simulink library "xpcseriallib"  (Simulink 7.7)
settings: Solver=FixedStepDiscrete  StartTime=0.0  StopTime=inf  RelTol=1e-3
undefined symbols (not defined in the file or in its folder): baddr1, baddr2, mbaseserialbinmask, mbaseserialmask, mdiamondemeraldfifomask, mdiamondemeraldmask, mmodemcontrol, mqua2mask, mquafifomask, mquamask, mrs232
libraries: xpcseriallib x614, xpclib x16, simulink x12
(part 2 of 7)

== system xpcseriallib/Diamond/Emerald-MM8  ==
  Diamond Emerald-MM8 Serial : Subsystem  InitFcn=mdiamondemeraldmask(4,8)  mask(RS232 Send Receive){group=Receive Setup, port=1, irqnum=5, saddr1=0x200, baud1=115200, parity1=None, ndata1=8, nstop1=1, fifomode1=16 deep, rlevel1=1, automode1=on, xmtfifosize1=1024, xmtdatatype1=8 bit uint null terminated, rcvfifosize1=1024, rcvmaxread1=1024, rcvminread1=1, rcvusedelim1=on, rcvdelim1=13, rcvdatatype1=count+16 bit uint, rcvsampletime1=-1, baud2=115200, parity2=None, ndata2=8, nstop2=1, fifomode2=16 deep, rlevel2=1, automode2=on, xmtfifosize2=1024, xmtdatatype2=8 bit uint null terminated, rcvfifosize2=1024, rcvmaxread2=1024, rcvminread2=1, rcvusedelim2=on, rcvdelim2=13, rcvdatatype2=count+16 bit uint, rcvsampletime2=-1, baud3=115200, parity3=None, ndata3=8, nstop3=1, fifomode3=16 deep, rlevel3=1, automode3=on, xmtfifosize3=1024, xmtdatatype3=8 bit uint null terminated, rcvfifosize3=1024, rcvmaxread3=1024, rcvminread3=1, rcvusedelim3=on, rcvdelim3=13, rcvdatatype3=count+16 bit uint, rcvsampletime3=-1, baud4=115200, parity4=None, ndata4=8, nstop4=1, fifomode4=16 deep, rlevel4=1, automode4=on, xmtfifosize4=1024, xmtdatatype4=8 bit uint null terminated, rcvfifosize4=1024, rcvmaxread4=1024, rcvminread4=1, rcvusedelim4=on, rcvdelim4=13, rcvdatatype4=count+16 bit uint, rcvsampletime4=-1, baud5=115200, parity5=None, ndata5=8, nstop5=1, fifomode5=16 deep, rlevel5=1, automode5=on, xmtfifosize5=1024, xmtdatatype5=8 bit uint null terminated, rcvfifosize5=1024, rcvmaxread5=1024, rcvminread5=1, rcvusedelim5=on, rcvdelim5=13, rcvdatatype5=count+16 bit uint, rcvsampletime5=-1, baud6=115200, parity6=None, ndata6=8, nstop6=1, fifomode6=16 deep, rlevel6=1, automode6=on, xmtfifosize6=1024, xmtdatatype6=8 bit uint null terminated, rcvfifosize6=1024, rcvmaxread6=1024, rcvminread6=1, rcvusedelim6=on, rcvdelim6=13, rcvdatatype6=count+16 bit uint, rcvsampletime6=-1, baud7=115200, parity7=None, ndata7=8, nstop7=1, fifomode7=16 deep, rlevel7=1, automode7=on, xmtfifosize7=1024, xmtdatatype7=8 bit uint null terminated, rcvfifosize7=1024, rcvmaxread7=1024, rcvminread7=1, rcvusedelim7=on, rcvdelim7=13, rcvdatatype7=count+16 bit uint, rcvsampletime7=-1, baud8=115200, parity8=None, ndata8=8, nstop8=1, fifomode8=16 deep, rlevel8=1, automode8=on, xmtfifosize8=1024, xmtdatatype8=8 bit uint null terminated, rcvfifosize8=1024, rcvmaxread8=1024, rcvminread8=1, rcvusedelim8=on, rcvdelim8=13, rcvdatatype8=count+16 bit uint, rcvsampletime8=-1}
      mask prompts: group "Parameter group:"; port "Port to modify:"; irqnum "IRQ number:"; saddr1 "Base address:"; baud1 "Baud rate:"; parity1 "Parity:"; ndata1 "Data bits:"; nstop1 "Stop bits:"; fifomode1 "Hardware FIFO size:"; rlevel1 "Receive FIFO interrupt level:"; automode1 "Auto RTS/CTS:"; xmtfifosize1 "Transmit software FIFO size:"; xmtdatatype1 "Transmit FIFO data type:"; rcvfifosize1 "Receive software FIFO size:"; rcvmaxread1 "Receive maximum read:"; rcvminread1 "Receive minimum read:"; rcvusedelim1 "Read to delimiter:"; rcvdelim1 "Delimiter:"; rcvdatatype1 "Receive data type:"; rcvsampletime1 "Receive SampleTime:"; baud2 "Baud rate:"; parity2 "Parity:"; ndata2 "Data bits:"; nstop2 "Stop bits:"; fifomode2 "Hardware FIFO size:"; rlevel2 "Receive FIFO interrupt level:"; automode2 "Auto RTS/CTS:"; xmtfifosize2 "Transmit software FIFO size:"; xmtdatatype2 "Transmit FIFO data type:"; rcvfifosize2 "Receive software FIFO size:"; rcvmaxread2 "Receive maximum read:"; rcvminread2 "Receive minimum read:"; rcvusedelim2 "Read to delimiter:"; rcvdelim2 "Delimiter:"; rcvdatatype2 "Receive data type:"; rcvsampletime2 "Receive SampleTime:"; baud3 "Baud rate:"; parity3 "Parity:"; ndata3 "Data bits:"; nstop3 "Stop bits:"; fifomode3 "Hardware FIFO size:"; rlevel3 "Receive FIFO interrupt level:"; automode3 "Auto RTS/CTS:"; xmtfifosize3 "Transmit software FIFO size:"; xmtdatatype3 "Transmit fifo data type:"; rcvfifosize3 "Receive software FIFO size:"; rcvmaxread3 "Receive maximum read:"; rcvminread3 "Receive minimum read:"; rcvusedelim3 "Read to delimiter:"; rcvdelim3 "Delimiter:"; rcvdatatype3 "Receive data type:"; rcvsampletime3 "Receive SampleTime:"; baud4 "Baud rate:"; parity4 "Parity:"; ndata4 "Data bits:"; nstop4 "Stop bits:"; fifomode4 "Hardware FIFO size:"; rlevel4 "Receive FIFO interrupt level:"; automode4 "Auto RTS/CTS:"; xmtfifosize4 "Transmit software FIFO size:"; xmtdatatype4 "Transmit FIFO data type:"; rcvfifosize4 "Receive software FIFO size:"; rcvmaxread4 "Receive maximum read:"; rcvminread4 "Receive minimum read:"; rcvusedelim4 "Read to delimiter:"; rcvdelim4 "Delimiter:"; rcvdatatype4 "Receive data type:"; rcvsampletime4 "Receive SampleTime:"; baud5 "Baud rate:"; parity5 "Parity:"; ndata5 "Data bits:"; nstop5 "Stop bits:"; fifomode5 "Hardware FIFO size:"; rlevel5 "Receive FIFO interrupt level:"; automode5 "Auto RTS/CTS:"; xmtfifosize5 "Transmit software FIFO size:"; xmtdatatype5 "Transmit FIFO data type:"; rcvfifosize5 "Receive software FIFO size:"; rcvmaxread5 "Receive maximum read:"; rcvminread5 "Receive minimum read:"; rcvusedelim5 "Read to delimiter:"; rcvdelim5 "Delimiter:"; rcvdatatype5 "Receive data type:"; rcvsampletime5 "Receive SampleTime:"; baud6 "Baud rate:"; parity6 "Parity:"; ndata6 "Data bits:"; nstop6 "Stop bits:"; fifomode6 "Hardware FIFO size:"; rlevel6 "Receive FIFO interrupt level:"; automode6 "Auto RTS/CTS:"; xmtfifosize6 "Transmit software FIFO size:"; xmtdatatype6 "Transmit FIFO data type:"; rcvfifosize6 "Receive software FIFO size:"; rcvmaxread6 "Receive maximum read:"; rcvminread6 "Receive minimum read:"; rcvusedelim6 "Read to delimiter:"; rcvdelim6 "Delimiter:"; rcvdatatype6 "Receive data type:"; rcvsampletime6 "Receive SampleTime:"; baud7 "Baud rate:"; parity7 "Parity:"; ndata7 "Data bits:"; nstop7 "Stop bits:"; fifomode7 "Hardware FIFO size:"; rlevel7 "Receive FIFO interrupt level:"; automode7 "Auto RTS/CTS:"; xmtfifosize7 "Transmit software FIFO size:"; xmtdatatype7 "Transmit FIFO data type:"; rcvfifosize7 "Receive software FIFO size:"; rcvmaxread7 "Receive maximum read:"; rcvminread7 "Receive minimum read:"; rcvusedelim7 "Read to delimiter:"; rcvdelim7 "Delimiter:"; rcvdatatype7 "Receive data type:"; rcvsampletime7 "Receive SampleTime:"; baud8 "Baud rate:"; parity8 "Parity:"; ndata8 "Data bits:"; nstop8 "Stop bits:"; fifomode8 "Hardware FIFO size:"; rlevel8 "Receive FIFO interrupt level:"; automode8 "Auto RTS/CTS:"; xmtfifosize8 "Transmit software FIFO size:"; xmtdatatype8 "Transmit FIFO data type:"; rcvfifosize8 "Receive software FIFO size:"; rcvmaxread8 "Receive maximum read:"; rcvminread8 "Receive minimum read:"; rcvusedelim8 "Read to delimiter:"; rcvdelim8 "Delimiter:"; rcvdatatype8 "Receive data type:"; rcvsampletime8 "Receive SampleTime:"
      mask help:
      | Diamond Emerald MM-8
      | RS232 Send Receive Subsystem
      mask init:
      | addr = mdiamondemeraldmask( 1, 8 );
      | % addr(1) is base address, not used
      | baddr1 = addr{2};
      | baddr2 = addr{3};
      | baddr3 = addr{4};
      | baddr4 = addr{5};
      | baddr5 = addr{6};
      | baddr6 = addr{7};
      | baddr7 = addr{8};
      | baddr8 = addr{9};
      | istat = addr{10};
      | mdiamondemeraldmask( 3, 8 );
      mask Help: helpview(fullfile(docroot, 'mapfiles', 'xpc.map'), 'Baseboard_Serial_Subsystem')
      mask StyleString: popup(Board Setup|Basic Setup|Transmit Setup|Receive Setup),popup(1|2|3|4|5|6|7|8),edit,popup(0x100|0x140|0x180|0x1c0|0x200|0x240|0x280|0x2c0|0x300|0x340|0x380|0x3c0),popup(115200|57600|38400|19200|9600|4800|2400|1200|600|300|110),popup(None|Even|Odd|Mark|Space),popup(5|6|7|8),popup(1|2),popup(64 deep|16 deep|1 deep),popup(1|quarter full|half full|almost full),checkbox,edit,popup(count+32 bit int|count+32 bit uint|count+16 bit int|count+16 bit uint|8 bit int null terminated|8 bit uint null terminated),edit,edit,edit,checkbox,edit,popup(count+32 bit int|count+32 bit uint|count+16 bit int|count+16 bit uint|8 bit int null terminated|8 bit uint null terminated),edit,popup(115200|57600|38400|19200|9600|4800|2400|1200|600|300|110),popup(None|Even|Odd|Mark|Space),popup(5|6|7|8),popup(1|2),popup(64 deep|16 deep|1 deep),popup(1|quarter full|half full|almost full),checkbox,edit,popup(count+32 bit int|count+32 bit uint|count+16 bit int|count+16 bit uint|8 bit int null terminated|8 bit uint null terminated),edit,edit,edit,checkbox,edit,popup(count+32 bit int|count+32 bit uint|count+16 bit int|count+16 bit uint|8 bit int null terminated|8 bit uint null terminated),edit,popup(115200|57600|38400|19200|9600|4800|2400|1200|600|300|110),popup(None|Even|Odd|Mark|Space),popup(5|6|7|8),popup(1|2),popup(64 deep|16 deep|1 deep),popup(1|quarter full|half full|almost full),checkbox,edit,popup(count+32 bit int|count+32 bit uint|count+16 bit int|count+16 bit uint|8 bit int null terminated|8 bit uint null terminated),edit,edit,edit,checkbox,edit,popup(count+32 bit int|count+32 bit uint|count+16 bit int|count+16 bit uint|8 bit int null terminated|8 bit uint null terminated),edit,popup(115200|57600|38400|19200|9600|4800|2400|1200|600|300|110),popup(None|Even|Odd|Mark|Space),popup(5|6|7|8),popup(1|2),popup(64 deep|16 deep|1 deep),popup(1|quarter full|half full|almost full),checkbox,edit,popup(count+32 bit int|count+32 bit uint|count+16 bit int|count+16 bit uint|8 bit int null terminated|8 bit uint null terminated),edit,edit,edit,checkbox,edit,popup(count+32 bit int|count+32 bit uint|count+16 bit int|count+16 bit uint|8 bit int null terminated|8 bit uint null terminated),edit,popup(115200|57600|38400|19200|9600|4800|2400|1200|600|300|110),popup(None|Even|Odd|Mark|Space),popup(5|6|7|8),popup(1|2),popup(64 deep|16 deep|1 deep),popup(1|quarter full|half full|almost full),checkbox,edit,popup(count+32 bit int|count+32 bit uint|count+16 bit int|count+16 bit uint|8 bit int null terminated|8 bit uint null terminated),edit,edit,edit,checkbox,edit,popup(count+32 bit int|count+32 bit uint|count+16 bit int|count+16 bit uint|8 bit int null terminated|8 bit uint null terminated),edit,popup(115200|57600|38400|19200|9600|4800|2400|1200|600|300|110),popup(None|Even|Odd|Mark|Space),popup(5|6|7|8),popup(1|2),popup(64 deep|16 deep|1 deep),popup(1|quarter full|half full|almost full),checkbox,edit,popup(count+32 bit int|count+32 bit uint|count+16 bit int|count+16 bit uint|8 bit int null terminated|8 bit uint null terminated),edit,edit,edit,checkbox,edit,popup(count+32 bit int|count+32 bit uint|count+16 bit int|count+16 bit uint|8 bit int null terminated|8 bit uint null terminated),edit,popup(115200|57600|38400|19200|9600|4800|2400|1200|600|300|110),popup(None|Even|Odd|Mark|Space),popup(5|6|7|8),popup(1|2),popup(64 deep|16 deep|1 deep),popup(1|quarter full|half full|almost full),checkbox,edit,popup(count+32 bit int|count+32 bit uint|count+16 bit int|count+16 bit uint|8 bit int null terminated|8 bit uint null terminated),edit,edit,edit,checkbox,edit,popup(count+32 bit int|count+32 bit uint|count+16 bit int|count+16 bit uint|8 bit int null terminated|8 bit uint null terminated),edit,popup(115200|57600|38400|19200|9600|4800|2400|1200|600|300|110),popup(None|Even|Odd|Mark|Space),popup(5|6|7|8),popup(1|2),popup(64 deep|16 deep|1 deep),popup(1|quarter full|half full|almost full),checkbox,edit,popup(count+32 bit int|count+32 bit uint|count+16 bit int|count+16 bit uint|8 bit int null terminated|8 bit uint null terminated),edit,edit,edit,checkbox,edit,popup(count+32 bit int|count+32 bit uint|count+16 bit int|count+16 bit uint|8 bit int null terminated|8 bit uint null terminated),edit
      mask CallbackString:
      | mdiamondemeraldmask( 2, 8 );
      | |mdiamondemeraldmask( 2, 8 );||||||||||||||||||||||||||||||||||||||||||||||||||||||||||||||||||||||||||||||||||||||||||||||||||||||||||||||||||||||||||||||||||
      mask Display:
      | disp('Diamond\n\nEmerald\n\nRS232\nSend Receive');
      | port_label('input',1,'XMT1');
      | port_label('input',2,'XMT2');
      | port_label('input',3,'XMT3');
      | port_label('input',4,'XMT4');
      | port_label('input',5,'XMT5');
      | port_label('input',6,'XMT6');
      | port_label('input',7,'XMT7');
      | port_label('input',8,'XMT8');
      | port_label('output',1,'RCV1');
      | port_label('output',2,'RCV2');
      | port_label('output',3,'RCV3');
      | port_label('output',4,'RCV4');
      | port_label('output',5,'RCV5');
      | port_label('output',6,'RCV6');
      | port_label('output',7,'RCV7');
      | port_label('output',8,'RCV8');
  Diamond Emerald-MM8 Serial F : Subsystem  InitFcn=mdiamondemeraldmask(4,8)  mask(RS232 Send Receive){group=Board Setup, port=1, irqnum=5, saddr1=0x200, baud1=115200, parity1=None, ndata1=8, nstop1=1, fifomode1=16 deep, rlevel1=1, automode1=on, xmtfifosize1=1024, xmtdatatype1=8 bit uint null terminated, rcvfifosize1=1024, baud2=115200, parity2=None, ndata2=8, nstop2=1, fifomode2=16 deep, rlevel2=1, automode2=on, xmtfifosize2=1024, xmtdatatype2=8 bit uint null terminated, rcvfifosize2=1024, baud3=115200, parity3=None, ndata3=8, nstop3=1, fifomode3=16 deep, rlevel3=1, automode3=on, xmtfifosize3=1024, xmtdatatype3=8 bit uint null terminated, rcvfifosize3=1024, baud4=115200, parity4=None, ndata4=8, nstop4=1, fifomode4=16 deep, rlevel4=1, automode4=on, xmtfifosize4=1024, xmtdatatype4=8 bit uint null terminated, rcvfifosize4=1024, baud5=115200, parity5=None, ndata5=8, nstop5=1, fifomode5=16 deep, rlevel5=1, automode5=on, xmtfifosize5=1024, xmtdatatype5=8 bit uint null terminated, rcvfifosize5=1024, baud6=115200, parity6=None, ndata6=8, nstop6=1, fifomode6=16 deep, rlevel6=1, automode6=on, xmtfifosize6=1024, xmtdatatype6=8 bit uint null terminated, rcvfifosize6=1024, baud7=115200, parity7=None, ndata7=8, nstop7=1, fifomode7=16 deep, rlevel7=1, automode7=on, xmtfifosize7=1024, xmtdatatype7=8 bit uint null terminated, rcvfifosize7=1024, baud8=115200, parity8=None, ndata8=8, nstop8=1, fifomode8=16 deep, rlevel8=1, automode8=on, xmtfifosize8=1024, xmtdatatype8=8 bit uint null terminated, rcvfifosize8=1024}
      mask prompts: group "Parameter group:"; port "Port to modify:"; irqnum "IRQ number:"; saddr1 "Base address:"; baud1 "Baud rate:"; parity1 "Parity:"; ndata1 "Data bits:"; nstop1 "Stop bits:"; fifomode1 "Hardware FIFO size:"; rlevel1 "Receive FIFO interrupt level:"; automode1 "Auto RTS/CTS:"; xmtfifosize1 "Transmit software FIFO size:"; xmtdatatype1 "Transmit FIFO data type:"; rcvfifosize1 "Receive software FIFO size:"; baud2 "Baud rate:"; parity2 "Parity:"; ndata2 "Data bits:"; nstop2 "Stop bits:"; fifomode2 "Hardware FIFO size:"; rlevel2 "Receive FIFO interrupt level:"; automode2 "Auto RTS/CTS:"; xmtfifosize2 "Transmit software FIFO size:"; xmtdatatype2 "Transmit FIFO data type:"; rcvfifosize2 "Receive software FIFO size:"; baud3 "Baud rate:"; parity3 "Parity:"; ndata3 "Data bits:"; nstop3 "Stop bits:"; fifomode3 "Hardware FIFO size:"; rlevel3 "Receive FIFO interrupt level:"; automode3 "Auto RTS/CTS:"; xmtfifosize3 "Transmit software FIFO size:"; xmtdatatype3 "Transmit fifo data type:"; rcvfifosize3 "Receive software FIFO size:"; baud4 "Baud rate:"; parity4 "Parity:"; ndata4 "Data bits:"; nstop4 "Stop bits:"; fifomode4 "Hardware FIFO size:"; rlevel4 "Receive FIFO interrupt level:"; automode4 "Auto RTS/CTS:"; xmtfifosize4 "Transmit software FIFO size:"; xmtdatatype4 "Transmit FIFO data type:"; rcvfifosize4 "Receive software FIFO size:"; baud5 "Baud rate:"; parity5 "Parity:"; ndata5 "Data bits:"; nstop5 "Stop bits:"; fifomode5 "Hardware FIFO size:"; rlevel5 "Receive FIFO interrupt level:"; automode5 "Auto RTS/CTS:"; xmtfifosize5 "Transmit software FIFO size:"; xmtdatatype5 "Transmit FIFO data type:"; rcvfifosize5 "Receive software FIFO size:"; baud6 "Baud rate:"; parity6 "Parity:"; ndata6 "Data bits:"; nstop6 "Stop bits:"; fifomode6 "Hardware FIFO size:"; rlevel6 "Receive FIFO interrupt level:"; automode6 "Auto RTS/CTS:"; xmtfifosize6 "Transmit software FIFO size:"; xmtdatatype6 "Transmit FIFO data type:"; rcvfifosize6 "Receive software FIFO size:"; baud7 "Baud rate:"; parity7 "Parity:"; ndata7 "Data bits:"; nstop7 "Stop bits:"; fifomode7 "Hardware FIFO size:"; rlevel7 "Receive FIFO interrupt level:"; automode7 "Auto RTS/CTS:"; xmtfifosize7 "Transmit software FIFO size:"; xmtdatatype7 "Transmit FIFO data type:"; rcvfifosize7 "Receive software FIFO size:"; baud8 "Baud rate:"; parity8 "Parity:"; ndata8 "Data bits:"; nstop8 "Stop bits:"; fifomode8 "Hardware FIFO size:"; rlevel8 "Receive FIFO interrupt level:"; automode8 "Auto RTS/CTS:"; xmtfifosize8 "Transmit software FIFO size:"; xmtdatatype8 "Transmit FIFO data type:"; rcvfifosize8 "Receive software FIFO size:"
      mask help:
      | Diamond Emerald MM-8
      | RS232 Send Receive Subsystem
      mask init:
      | addr = mdiamondemeraldfifomask( 1, 8 );
      | % addr(1) is base address, not used
      | baddr1 = addr{2};
      | baddr2 = addr{3};
      | baddr3 = addr{4};
      | baddr4 = addr{5};
      | baddr5 = addr{6};
      | baddr6 = addr{7};
      | baddr7 = addr{8};
      | baddr8 = addr{9};
      | istat = addr{10};
      | mdiamondemeraldfifomask( 3, 8 );
      mask Help: helpview(fullfile(docroot, 'mapfiles', 'xpc.map'), 'Baseboard_Serial_Subsystem')
      mask StyleString: popup(Board Setup|Basic Setup|FIFO Setup),popup(1|2|3|4|5|6|7|8),edit,popup(0x100|0x140|0x180|0x1c0|0x200|0x240|0x280|0x2c0|0x300|0x340|0x380|0x3c0),popup(115200|57600|38400|19200|9600|4800|2400|1200|600|300|110),popup(None|Even|Odd|Mark|Space),popup(5|6|7|8),popup(1|2),popup(64 deep|16 deep|1 deep),popup(1|quarter full|half full|almost full),checkbox,edit,popup(count+32 bit int|count+32 bit uint|count+16 bit int|count+16 bit uint|8 bit int null terminated|8 bit uint null terminated),edit,popup(115200|57600|38400|19200|9600|4800|2400|1200|600|300|110),popup(None|Even|Odd|Mark|Space),popup(5|6|7|8),popup(1|2),popup(64 deep|16 deep|1 deep),popup(1|quarter full|half full|almost full),checkbox,edit,popup(count+32 bit int|count+32 bit uint|count+16 bit int|count+16 bit uint|8 bit int null terminated|8 bit uint null terminated),edit,popup(115200|57600|38400|19200|9600|4800|2400|1200|600|300|110),popup(None|Even|Odd|Mark|Space),popup(5|6|7|8),popup(1|2),popup(64 deep|16 deep|1 deep),popup(1|quarter full|half full|almost full),checkbox,edit,popup(count+32 bit int|count+32 bit uint|count+16 bit int|count+16 bit uint|8 bit int null terminated|8 bit uint null terminated),edit,popup(115200|57600|38400|19200|9600|4800|2400|1200|600|300|110),popup(None|Even|Odd|Mark|Space),popup(5|6|7|8),popup(1|2),popup(64 deep|16 deep|1 deep),popup(1|quarter full|half full|almost full),checkbox,edit,popup(count+32 bit int|count+32 bit uint|count+16 bit int|count+16 bit uint|8 bit int null terminated|8 bit uint null terminated),edit,popup(115200|57600|38400|19200|9600|4800|2400|1200|600|300|110),popup(None|Even|Odd|Mark|Space),popup(5|6|7|8),popup(1|2),popup(64 deep|16 deep|1 deep),popup(1|quarter full|half full|almost full),checkbox,edit,popup(count+32 bit int|count+32 bit uint|count+16 bit int|count+16 bit uint|8 bit int null terminated|8 bit uint null terminated),edit,popup(115200|57600|38400|19200|9600|4800|2400|1200|600|300|110),popup(None|Even|Odd|Mark|Space),popup(5|6|7|8),popup(1|2),popup(64 deep|16 deep|1 deep),popup(1|quarter full|half full|almost full),checkbox,edit,popup(count+32 bit int|count+32 bit uint|count+16 bit int|count+16 bit uint|8 bit int null terminated|8 bit uint null terminated),edit,popup(115200|57600|38400|19200|9600|4800|2400|1200|600|300|110),popup(None|Even|Odd|Mark|Space),popup(5|6|7|8),popup(1|2),popup(64 deep|16 deep|1 deep),popup(1|quarter full|half full|almost full),checkbox,edit,popup(count+32 bit int|count+32 bit uint|count+16 bit int|count+16 bit uint|8 bit int null terminated|8 bit uint null terminated),edit,popup(115200|57600|38400|19200|9600|4800|2400|1200|600|300|110),popup(None|Even|Odd|Mark|Space),popup(5|6|7|8),popup(1|2),popup(64 deep|16 deep|1 deep),popup(1|quarter full|half full|almost full),checkbox,edit,popup(count+32 bit int|count+32 bit uint|count+16 bit int|count+16 bit uint|8 bit int null terminated|8 bit uint null terminated),edit
      mask CallbackString:
      | mdiamondemeraldfifomask( 2, 8 );
      | |mdiamondemeraldfifomask( 2, 8 );||||||||||||||||||||||||||||||||||||||||||||||||||||||||||||||||||||||||||||||||||
      mask Display:
      | disp('Diamond\n\nEmerald\n\nRS232\n\nSend Receive\n\nFIFO OUT');
      | port_label('input',1,'XMT1');
      | port_label('input',2,'XMT2');
      | port_label('input',3,'XMT3');
      | port_label('input',4,'XMT4');
      | port_label('input',5,'XMT5');
      | port_label('input',6,'XMT6');
      | port_label('input',7,'XMT7');
      | port_label('input',8,'XMT8');
      | port_label('output',1,'FIFO1');
      | port_label('output',2,'FIFO2');
      | port_label('output',3,'FIFO3');
      | port_label('output',4,'FIFO4');
      | port_label('output',5,'FIFO5');
      | port_label('output',6,'FIFO6');
      | port_label('output',7,'FIFO7');
      | port_label('output',8,'FIFO8');
  "Diamond Emerald-MM8 " : Subsystem
  "Modem Control " : S-Function  InitFcn=mmodemcontrol(5);  FunctionName=modemcontrolemeraldmm  Parameters=addr, boardtype, rts, dtr, count  EnableBusSupport=off  mask(Modem Control){port=1, rts=on, dtr=on, firstaddr=0x200}
      mask prompts: firstaddr "Configuration port address:"
      mask help:
      | Diamond Emerald-MM-8
      | Modem Control
      mask init:
      | count = 0;
      | boardtype = 6;
      | [maskdisplay, count, addr] = mmodemcontrol( 2, rts, dtr, boardtype, port, firstaddr );
      | addr = hex2dec( addr(3:end) );
      | set_param( gcb, 'MaskDisplay', maskdisplay );
      mask Help: helpview(fullfile(docroot, 'mapfiles', 'xpc.map'), 'Emerald_MODEM_Control')
      mask StyleString: popup(1|2|3|4|5|6|7|8),checkbox,checkbox,popup(0x100|0x140|0x180|0x1c0|0x200|0x240|0x280|0x2c0|0x300|0x340|0x380|0x3c0)
      mask Display: disp('Diamond\nEmerald-MM-8\nModem Control');port_label('input',1,'RTS');port_label('input',2,'DTR');
  "Modem Status " : S-Function  FunctionName=modemstatusemeraldmm  Parameters=addr, boardtype, cts, dsr, ring, dcd, count, sampletime  EnableBusSupport=off  mask(Modem Status){port=1, cts=on, dsr=on, ring=on, dcd=on, sampletime=-1, firstaddr=0x200}
      mask prompts: ring "RI:"; firstaddr "Configuration port address:"
      mask help:
      | Diamond Emerald-MM-8
      | Modem Status
      mask init:
      | count = 0;
      | boardtype = 6;
      | [maskdisplay, count, addr] = mmodemstatus( 2, cts, dsr, ring, dcd, boardtype, port, firstaddr );
      | addr = hex2dec( addr(3:end) );
      | set_param( gcb, 'MaskDisplay', maskdisplay );
      mask Help: helpview(fullfile(docroot, 'mapfiles', 'xpc.map'), 'Emerald_MODEM_Status')
      mask StyleString: popup(1|2|3|4|5|6|7|8),checkbox,checkbox,checkbox,checkbox,edit,popup(0x100|0x140|0x180|0x1c0|0x200|0x240|0x280|0x2c0|0x300|0x340|0x380|0x3c0)
      mask Display: disp('Diamond\nEmerald-MM-8\nModem Status');port_label('output',1,'CTS');port_label('output',2,'DSR');port_label('output',3,'RI');port_label('output',4,'DCD');

== system xpcseriallib/Mainboard/Baseboard Serial ==
  In1 : Inport
  In2 : Inport  Port=2
  Enable TX 1 : xpcseriallib/Mainboard/Baseboard Serial Internal  blocks/Enable TX   addr=baddr1
  Enable TX 2 : xpcseriallib/Mainboard/Baseboard Serial Internal  blocks/Enable TX   addr=baddr2
  FIFO read 1 : xpcseriallib/FIFO read   maxsize=1024  minsize=1  usedelimiter=on  delimiter=13  outputtype=count+16 bit uint  enable=off  enableout=off  sampletime=.01
  FIFO read 2 : xpcseriallib/FIFO read   maxsize=1024  minsize=1  usedelimiter=on  delimiter=13  outputtype=count+16 bit uint  enable=off  enableout=off  sampletime=.01
  FIFO write 1 : xpcseriallib/FIFO write   size=1024  inputtype=8 bit uint null terminated  present=on  sampletime=-1  id=XMT channel 1, IRQ 4
  FIFO write 2 : xpcseriallib/FIFO write   size=1024  inputtype=8 bit uint null terminated  present=on  sampletime=-1  id=XMT channel 2, IRQ 4
  IRQ Source : xpclib/Asynchronous Event/IRQ Source  irqNo=4  preempt=10  b_type=None/Other  slot=-1
  RS232 ISR : Subsystem  TreatAsAtomicUnit=on  mask(RS232 ISR){addr1=baddr1, addr2=baddr2}
      mask prompts: addr1 "First channel address:"; addr2 "Second channel address:"
      mask help:
      | Baseboard Serial
      | Interrupt Service Routine
      mask init:
      | baddr1 = addr1;
      | baddr2 = addr2;
      mask Display:
      | disp('Baseboard\nSerial\nISR');
      | port_label('input', 1, 'XMT1');
      | port_label('input', 2, 'XMT3');
      | port_label('output', 1, 'RCV1');
      | port_label('output', 2, 'RCV3');
  Rate Transition{,1..3} (4 alike) : RateTransition  Integrity=off  Deterministic=off
  Setup1 : xpcseriallib/Mainboard/Baseboard Serial Internal  blocks/Setup  baud=115200  width=8  nstop=1  parity=None  fmode=16 deep  rlevel=half full  ctsmode=off  addr=baddr1
  Setup2 : xpcseriallib/Mainboard/Baseboard Serial Internal  blocks/Setup  baud=115200  width=8  nstop=1  parity=None  fmode=16 deep  rlevel=half full  ctsmode=off  addr=baddr2
  Out1 : Outport
  Out2 : Outport  Port=2
  wires:
  RS232 ISR/2(Recv 2) -> Rate Transition3/1
  RS232 ISR/1(Recv 1) -> Rate Transition1/1
  Rate Transition/1 -> RS232 ISR/1(Xmt 1)
  Rate Transition2/1 -> RS232 ISR/2(Xmt 2)
  FIFO write 2/2 -> Enable TX 2/1
  FIFO read 2/1 -> Out2/1
  Rate Transition3/1 -> FIFO read 2/1
  FIFO read 1/1 -> Out1/1
  Rate Transition1/1 -> FIFO read 1/1
  In2/1 -> FIFO write 2/1
  FIFO write 2/1 -> Rate Transition2/1
  In1/1 -> FIFO write 1/1
  FIFO write 1/1 -> Rate Transition/1
  IRQ Source/1 -> RS232 ISR/Trigger
  FIFO write 1/2 -> Enable TX 1/1

== system xpcseriallib/Mainboard/Baseboard Serial Internal  blocks ==
  "Enable TX " : S-Function  FunctionName=sertxenablebase  Parameters=addr  EnableBusSupport=off  mask(Enable TX Int){addr=0}
      mask prompts: addr "Base address:"
      mask help:
      | Baseboard Serial
      | Enable TX Interrupt
      mask init:
      | addr = hex2dec( addr(3:end) );
      mask Help: helpview(fullfile(docroot, 'mapfiles', 'xpc.map'), 'Baseboard_Enable_Int')
      mask Display:
      | disp('Baseboard\nSerial\nEnable TX Int');
      | port_label('input', 1, 'E');
  Filter Int Reason : S-Function  FunctionName=filterserint  Parameters=port, value  EnableBusSupport=off  mask(Interrupt Source Filter){port=1, value=Receive data}
      mask prompts: value "Filter value:"
      mask help:
      | Baseboard
      | Interrupt Source Filter
      mask Help: helpview(fullfile(docroot, 'mapfiles', 'xpc.map'), 'Baseboard_Filter_Ints')
      mask StyleString: popup(1|2),popup(Receive data|Transmitter empty|Modem status change)
      mask Display:
      | disp('Baseboard\nSerial\nFilter Int Reason');
      | port_label('input', 1, 'S' );
      | port_label('output', 1, 'E' );
  Read HW FIFO : S-Function  FunctionName=serreadbase  Parameters=addr, flush  EnableBusSupport=off  mask(Read Data Port){flush=on, addr=0}
      mask prompts: flush "Flush HW FIFO on startup"; addr "Base address:"
      mask help:
      | Baseboard
      | Read Data Port
      mask init:
      | addr = hex2dec( addr(3:end) );
      mask Help: helpview(fullfile(docroot, 'mapfiles', 'xpc.map'), 'Baseboard_Read_HW')
      mask Display:
      | disp('Baseboard\nSerial\nRead HW FIFO');
      | port_label('input', 1, 'E');
      | port_label('output', 1, 'D');
  Read Int Status FC : S-Function  FunctionName=iquerybase  Parameters=addr1, addr2  EnableBusSupport=off  mask(Interrupt Query){addr1=baddr1, addr2=baddr2}
      mask prompts: addr1 "Base address 1"; addr2 "Base address 2"
      mask help:
      | Baseboard Serial
      | Interrupt Query
      mask init:
      | addr1 = hex2dec( addr1(3:end) );
      | addr2 = hex2dec( addr2(3:end) );
      mask Help: helpview(fullfile(docroot, 'mapfiles', 'xpc.map'), 'Baseboard_Interrupt_Query')
      mask Display:
      | disp('Baseboard\nSerial\nDispatch Int Status');
      | port_label('output', 1, 'FC' );
      | port_label('output', 2, 'D' );
  Setup : S-Function  FunctionName=sersetupbase  Parameters=addr, baud, width, nstop, parity, fmode, ctsmode, rlevel  EnableBusSupport=off  mask(setup){baud=115200, width=8, nstop=1, parity=None, fmode=16 deep, rlevel=half full, ctsmode=off, addr=0}
      mask prompts: baud "Baud rate:"; width "Number of data bits:"; nstop "Number of stop bits:"; fmode "FIFO mode:"; rlevel "Receive trigger level:"; ctsmode "Enable auto RTS/CTS"; addr "Base Address:"
      mask help:
      | Baseboard
      | Serial
      | Setup
      mask init:
      | addr = hex2dec( addr(3:end) );
      mask Help: helpview(fullfile(docroot, 'mapfiles', 'xpc.map'), 'Baseboard_Setup')
      mask StyleString: popup(115200|57600|38400|19200|9600|4800|2400|1200|600|300|110),popup(5|6|7|8),popup(1|2),popup(None|Even|Odd|Mark|Space),popup(64 deep|16 deep|1 deep),popup(1|quarter full|half full|almost full),checkbox,edit
      mask Display: disp('Baseboard\nSerial\nSetup');
  Write HW FIFO : S-Function  FunctionName=serwritebase  Parameters=addr  EnableBusSupport=off  mask(Write Data Port){addr=0}
      mask prompts: addr "Base address:"
      mask help:
      | Baseboard
      | Write Data Port
      mask init:
      | addr = hex2dec( addr(3:end) );
      mask Help: helpview(fullfile(docroot, 'mapfiles', 'xpc.map'), 'Baseboard_Write_HW')
      mask Display:
      | disp('Baseboard\nSerial\nWrite HW FIFO');
      | port_label('input', 1, 'D');
      | port_label('input', 2, 'E');

== system xpcseriallib/Mainboard/Baseboard Serial F ==
  In1 : Inport
  In2 : Inport  Port=2
  Enable TX 1 : xpcseriallib/Mainboard/Baseboard Serial Internal  blocks/Enable TX   addr=baddr1
  Enable TX 2 : xpcseriallib/Mainboard/Baseboard Serial Internal  blocks/Enable TX   addr=baddr2
  FIFO write 1 : xpcseriallib/FIFO write   size=1024  inputtype=8 bit uint null terminated  present=on  sampletime=-1  id=XMT channel 1, IRQ 4
  FIFO write 2 : xpcseriallib/FIFO write   size=1024  inputtype=8 bit uint null terminated  present=on  sampletime=-1  id=XMT channel 2, IRQ 4
  IRQ Source : xpclib/Asynchronous Event/IRQ Source  irqNo=4  preempt=10  b_type=None/Other  slot=-1
  RS232 ISR : Subsystem  TreatAsAtomicUnit=on  mask(RS232 ISR){addr1=baddr1, addr2=baddr2}
      mask prompts: addr1 "First channel address:"; addr2 "Second channel address:"
      mask help:
      | Baseboard Serial
      | Interrupt Service Routine
      mask init:
      | baddr1 = addr1;
      | baddr2 = addr2;
      mask Display:
      | disp('Baseboard\nSerial\nISR');
      | port_label('input', 1, 'XMT1');
      | port_label('input', 2, 'XMT3');
      | port_label('output', 1, 'RCV1');
      | port_label('output', 2, 'RCV3');
  Rate Transition{,1..3} (4 alike) : RateTransition  Integrity=off  Deterministic=off
  Setup1 : xpcseriallib/Mainboard/Baseboard Serial Internal  blocks/Setup  baud=115200  width=8  nstop=1  parity=None  fmode=16 deep  rlevel=half full  ctsmode=off  addr=baddr1
  Setup2 : xpcseriallib/Mainboard/Baseboard Serial Internal  blocks/Setup  baud=115200  width=8  nstop=1  parity=None  fmode=16 deep  rlevel=half full  ctsmode=off  addr=baddr2
  Out1 : Outport
  Out2 : Outport  Port=2
  wires:
  Rate Transition2/1 -> RS232 ISR/2(Xmt 2)
  FIFO write 2/2 -> Enable TX 2/1
  Rate Transition3/1 -> Out2/1
  Rate Transition1/1 -> Out1/1
  In2/1 -> FIFO write 2/1
  FIFO write 2/1 -> Rate Transition2/1
  In1/1 -> FIFO write 1/1
  FIFO write 1/1 -> Rate Transition/1
  RS232 ISR/2(Recv 2) -> Rate Transition3/1
  RS232 ISR/1(Recv 1) -> Rate Transition1/1
  Rate Transition/1 -> RS232 ISR/1(Xmt 1)
  IRQ Source/1 -> RS232 ISR/Trigger
  FIFO write 1/2 -> Enable TX 1/1

== system xpcseriallib/Obsolete/Asynchronous Mode ==
  RS232 Receive : S-Function  FunctionName=rs232rec  Parameters=port, outStr, outport, numoutports, formatrecinfo, dtypes, ts, numeom  EnableBusSupport=off  mask(rs232rec){port=COM1, blockvar=[], ts=0.1}
      mask prompts: blockvar "Message struct name:"; ts "Sample time:"
      mask help:
      | RS-232 Mainboard Receive
      | Backward compatible for old models
      | Not for use in new models
      mask init:
      | inStr = '';
      | outStr = '';
      | [inStr,outStr,dtypes,maskdisplay,maskdescription,inport,outport, numinports, numoutports, formatsendinfo, formatrecinfo, waitarg, numeom] = mrs232 (1, blockvar, 1);
      | 
      | 
      | set_param(gcb,'MaskDisplay',maskdisplay);
      | %set_param(gcb,'MaskDescription',maskdescription);
      mask Help: helpview(fullfile(docroot, 'mapfiles', 'xpc.map'), 'RS232_Asynchronous-Mode_RS232-1')
      mask StyleString: popup(COM1|COM2|COM3|COM4),edit,edit
      mask Display: disp('RS-232\nMainboard\nReceive');
  RS232 Send : S-Function  FunctionName=rs232send  Parameters=port, inStr, inport, numinports, formatsendinfo, ts, waitarg  EnableBusSupport=off  mask(rs232send){port=COM1, blockvar=[], ts=0.1}
      mask prompts: blockvar "Message struct name:"; ts "Sample time:"
      mask help:
      | RS-232 Mainboard Send
      | Backward compatible for old models
      | Not for use in new models
      mask init:
      | inStr = '';
      | outStr = '';
      | [inStr,outStr,dtypes,maskdisplay,maskdescription,inport,outport, numinports, numoutports, formatsendinfo, formatrecinfo, waitarg] = mrs232 (1, blockvar, 2);
      | set_param(gcb,'MaskDisplay',maskdisplay);
      mask Help: helpview(fullfile(docroot, 'mapfiles', 'xpc.map'), 'RS232_Asynchronous-Mode_RS232')
      mask StyleString: popup(COM1|COM2|COM3|COM4),edit,edit
      mask Display: disp('RS-232\nMainboard\nSend');

== system xpcseriallib/Obsolete/Binary Mode ==
  Pack : xpclib/UDP/Pack  datatypes={'double'}  byteAlign=1
  RS232 Binary Receive : S-Function  FunctionName=rs232brec  Parameters=port,width,samptime  EnableBusSupport=off  mask(rs232brec){port=COM1, width=1, samptime=-1}
      mask prompts: port "COM port:"; width "Maximum width per packet:"; samptime "Sample time:"
      mask help:
      | RS232 Binary receive
      | Backward compatible for old models
      | Not for use in new models
      mask Help: helpview(fullfile(docroot, 'mapfiles', 'xpc.map'), 'RS232_Binary-Mode_RS232-Binary-Receive')
      mask StyleString: popup(COM1|COM2|COM3|COM4),edit,edit
      mask Display: port_label('input',  1, 'Length');port_label('input',  2, 'Enable');port_label('output', 1, 'Done');port_label('output', 2, 'Data');disp(sprintf('RS232 Receive\nCOM%d', port));
  RS232 Binary Send : S-Function  FunctionName=rs232bsend  Parameters=port,width,samptime  EnableBusSupport=off  mask(rs232bsend){port=COM1, width=1, samptime=-1}
      mask prompts: port "COM port:"; width "Maximum width per packet:"; samptime "Sample time:"
      mask help:
      | RS232 Binary send
      | Backward compatible for old models
      | Not for use in new models
      mask Help: helpview(fullfile(docroot, 'mapfiles', 'xpc.map'), 'RS232_Binary-Mode_RS232-Binary-Send')
      mask StyleString: popup(COM1|COM2|COM3|COM4),edit,edit
      mask Display: disp(sprintf('RS232 Send\nCOM%d', port));
  Unpack : xpclib/UDP/Unpack  dimensions={[1]}  datatypes={'double'}  byteAlign=1

== system xpcseriallib/Obsolete/Synchronous Mode ==
  RS232 SR : S-Function  FunctionName=rs232sendrec  Parameters=port, inStr, outStr, inport, outport, numinports, numoutports, formatsendinfo, formatrecinfo, waitarg, dtypes, ts, numeom, timeoutarg  EnableBusSupport=off  mask(rs232sendrec){port=COM1, blockvar=[], ts=0.1}
      mask prompts: blockvar "Message struct name:"; ts "Sample time:"
      mask help:
      | RS-232 Mainboard Send/Receive
      | Backward compatible for old models
      | Not for use in new models
      mask init:
      | inStr = '';
      | outStr = '';
      | [inStr,outStr,dtypes,maskdisplay,maskdescription,inport,outport, numinports, numoutports, formatsendinfo, formatrecinfo, waitarg, numeom, timeoutarg] = mrs232 (1, blockvar, 3);
      | set_param(gcb,'MaskDisplay',maskdisplay);
      mask Help: helpview(fullfile(docroot, 'mapfiles', 'xpc.map'), 'RS232_Synchronous-Mode_RS232')
      mask StyleString: popup(COM1|COM2|COM3|COM4),edit,edit
      mask Display: disp('RS-232\nMainboard\nSend/Receive');

== system xpcseriallib/Obsolete V 1.0/Asynchronous Mode ==
  "Receive " : Subsystem  mask(rs232rec){port=COM2, formatrec='start,%f,stop;', numb=1, ts=0.01}
      mask prompts: formatrec "Receive format:"; numb "Number of end-of-message characters:"; ts "Sample time:"
      mask help:
      | Version 1.0 compatible
      | RS-232 Mainboard Receive
      | Backward compatible for old models
      | Not for use in new models
      mask Help: helpview(fullfile(docroot, 'mapfiles', 'xpc.map'), 'RS232_Asynchronous-Mode_Receive')
      mask StyleString: popup(COM1|COM2|COM3|COM4),edit,edit,edit
      mask Display: disp('RS232\nMainboard\nReceive');
  "Send " : Subsystem  mask(rs232send){port=COM2, formatsend='start,%f,stop;', wait=off, ts=0.01}
      mask prompts: formatsend "Send format:"; wait "Wait until message is transmitted"; ts "Sample time:"
      mask help:
      | Version 1.0 compatible
      | RS-232 Mainboard Send
      | Backward compatible for old models
      | Not for use in new models
      mask Help: helpview(fullfile(docroot, 'mapfiles', 'xpc.map'), 'RS232_Asynchronous-Mode_Send')
      mask StyleString: popup(COM1|COM2|COM3|COM4),edit,checkbox,edit
      mask Display: disp('RS232\nMainboard\nSend');

== system xpcseriallib/Obsolete V 1.0/Setup  ==
  S-Function : S-Function  FunctionName=rs232_setup  Parameters=port,baudrate,databit, stopbit, parity, protocol, sendbuf, recbuf, 0  EnableBusSupport=off

== system xpcseriallib/Obsolete V 1.0/Synchronous Mode ==
  "Send & Receive " : Subsystem  mask(rs232sendrec){port=COM2, formatsend='start,%f,stop;', formatrec='start,%f,stop;', numb=1, ts=0.01}
      mask prompts: formatsend "Send format:"; formatrec "Receive format:"; numb "Number of end-of-message characters:"; ts "Sample time:"
      mask help:
      | Version 1.0 compatible Mainboard Send/Receive
      | Backward compatible for old models
      | Not for use in new models
      mask Help: helpview(fullfile(docroot, 'mapfiles', 'xpc.map'), 'RS232_Synchronous-Mode_Send-&-Receive')
      mask StyleString: popup(COM1|COM2|COM3|COM4),edit,edit,edit,edit
      mask Display: disp('RS232\nMainboard\nSend/Receive');

== system xpcseriallib/Quatech/DSCP-200/300 ==
  DSCP-200/300 Internal  blocks : Subsystem
  "DSCP-200/300 " : Subsystem  InitFcn=mqua2mask(3)  mask(RS422/485 Send Receive){group=Board Setup, port=1, irqnum=7, slot=-1, baud1=115200, parity1=None, ndata1=8, nstop1=1, fifomode1=64 deep, rlevel1=half full, onxmt1=None, xmtfifosize1=1024, xmtdatatype1=8 bit uint null terminated, rcvfifosize1=1024, rcvmaxread1=1024, rcvminread1=1, rcvusedelim1=on, rcvdelim1=13, rcvdatatype1=count+16 bit uint, rcvsampletime1=-1, baud2=115200, parity2=None, ndata2=8, nstop2=1, fifomode2=64 deep, rlevel2=half full, onxmt2=None, xmtfifosize2=1024, xmtdatatype2=8 bit uint null terminated, rcvfifosize2=1024, rcvmaxread2=1024, rcvminread2=1, rcvusedelim2=on, rcvdelim2=13, rcvdatatype2=count+16 bit uint, rcvsampletime2=-1}
      mask prompts: group "Parameter group:"; port "Port to modify:"; irqnum "IRQ number:"; baud1 "Baud rate:"; parity1 "Parity:"; ndata1 "Data bits:"; nstop1 "Stop bits:"; fifomode1 "Hardware FIFO size:"; rlevel1 "Receive FIFO interrupt level:"; onxmt1 "Assert on transmit:"; xmtfifosize1 "Transmit software FIFO size:"; xmtdatatype1 "Transmit FIFO data type:"; rcvfifosize1 "Receive software FIFO size:"; rcvmaxread1 "Receive maximum read:"; rcvminread1 "Receive minimum read:"; rcvusedelim1 "Read to delimiter:"; rcvdelim1 "Delimiter:"; rcvdatatype1 "Receive data type:"; rcvsampletime1 "Receive SampleTime:"; baud2 "Baud rate:"; parity2 "Parity:"; ndata2 "Data bits:"; nstop2 "Stop bits:"; fifomode2 "Hardware FIFO size:"; rlevel2 "Receive FIFO interrupt level:"; onxmt2 "Assert on transmit:"; xmtfifosize2 "Transmit software FIFO size:"; xmtdatatype2 "Transmit FIFO data type:"; rcvfifosize2 "Receive software FIFO size:"; rcvmaxread2 "Receive maximum read:"; rcvminread2 "Receive minimum read:"; rcvusedelim2 "Read to delimiter:"; rcvdelim2 "Delimiter:"; rcvdatatype2 "Receive data type:"; rcvsampletime2 "Receive SampleTime:"
      mask help:
      | DSCP-200/300
      | Quatech
      | RS422/485 Send Receive Subsystem
      mask init:
      | brdslot = slot;
      | mqua2mask( 1, 2 );
      mask Help: helpview(fullfile(docroot, 'mapfiles', 'xpc.map'), 'Quatech_Subsystem')
      mask StyleString: popup(Board Setup|Basic Setup|Transmit Setup|Receive Setup),popup(1|2),edit,edit,popup(921600|460800|230400|115200|57600|38400|19200|9600|4800|2400|1200|600|300|110),popup(None|Even|Odd|Mark|Space),popup(5|6|7|8),popup(1|2),popup(64 deep|16 deep|1 deep),popup(1|quarter full|half full|almost full),popup(None|RTS|DTR),edit,popup(count+32 bit int|count+32 bit uint|count+16 bit int|count+16 bit uint|8 bit int null terminated|8 bit uint null terminated),edit,edit,edit,checkbox,edit,popup(count+32 bit int|count+32 bit uint|count+16 bit int|count+16 bit uint|8 bit int null terminated|8 bit uint null terminated),edit,popup(921600|460800|230400|115200|57600|38400|19200|9600|4800|2400|1200|600|300|110),popup(None|Even|Odd|Mark|Space),popup(5|6|7|8),popup(1|2),popup(64 deep|16 deep|1 deep),popup(1|quarter full|half full|almost full),popup(None|RTS|DTR),edit,popup(count+32 bit int|count+32 bit uint|count+16 bit int|count+16 bit uint|8 bit int null terminated|8 bit uint null terminated),edit,edit,edit,checkbox,edit,popup(count+32 bit int|count+32 bit uint|count+16 bit int|count+16 bit uint|8 bit int null terminated|8 bit uint null terminated),edit
      mask CallbackString:
      | mqua2mask( 2, 2 );
      | |mqua2mask( 2, 2 );||||||||||||||||||||||||||||||||||
      mask Display:
      | disp('DSCP-200/300\nRS422/485\nSend Receive');
      | port_label( 'input', 1, 'XMT1' );
      | port_label( 'input', 2, 'XMT2' );
      | port_label( 'output', 1, 'RCV1' );
      | port_label( 'output', 2, 'RCV2' );
  DSCP-200/300 F : Subsystem  InitFcn=mquafifomask(3)  mask(RS422/485 Send Receive){group=Board Setup, port=1, irqnum=7, slot=-1, baud1=115200, parity1=None, ndata1=8, nstop1=1, fifomode1=64 deep, rlevel1=half full, onxmt1=None, xmtfifosize1=1024, xmtdatatype1=8 bit uint null terminated, rcvfifosize1=1024, baud2=115200, parity2=None, ndata2=8, nstop2=1, fifomode2=64 deep, rlevel2=half full, onxmt2=None, xmtfifosize2=1024, xmtdatatype2=8 bit uint null terminated, rcvfifosize2=1024}
      mask prompts: group "Parameter group:"; port "Port to modify:"; irqnum "IRQ number:"; baud1 "Baud rate:"; parity1 "Parity:"; ndata1 "Data bits:"; nstop1 "Stop bits:"; fifomode1 "Hardware FIFO size:"; rlevel1 "Receive FIFO interrupt level:"; onxmt1 "Assert on transmit:"; xmtfifosize1 "Transmit software FIFO size:"; xmtdatatype1 "Transmit FIFO data type:"; rcvfifosize1 "Receive software FIFO size:"; baud2 "Baud rate:"; parity2 "Parity:"; ndata2 "Data bits:"; nstop2 "Stop bits:"; fifomode2 "Hardware FIFO size:"; rlevel2 "Receive FIFO interrupt level:"; onxmt2 "Assert on transmit:"; xmtfifosize2 "Transmit software FIFO size:"; xmtdatatype2 "Transmit FIFO data type:"; rcvfifosize2 "Receive software FIFO size:"
      mask help:
      | DSCP-200/300
      | Quatech
      | RS422/485 Send Receive Subsystem
      mask init:
      | brdslot = slot;
      | mquafifomask( 1, 2, 2 );
      mask Help: helpview(fullfile(docroot, 'mapfiles', 'xpc.map'), 'Quatech_Subsystem')
      mask StyleString: popup(Board Setup|Basic Setup|FIFO Setup),popup(1|2),edit,edit,popup(921600|460800|230400|115200|57600|38400|19200|9600|4800|2400|1200|600|300|110),popup(None|Even|Odd|Mark|Space),popup(5|6|7|8),popup(1|2),popup(64 deep|16 deep|1 deep),popup(1|quarter full|half full|almost full),popup(None|RTS|DTR),edit,popup(count+32 bit int|count+32 bit uint|count+16 bit int|count+16 bit uint|8 bit int null terminated|8 bit uint null terminated),edit,popup(921600|460800|230400|115200|57600|38400|19200|9600|4800|2400|1200|600|300|110),popup(None|Even|Odd|Mark|Space),popup(5|6|7|8),popup(1|2),popup(64 deep|16 deep|1 deep),popup(1|quarter full|half full|almost full),popup(None|RTS|DTR),edit,popup(count+32 bit int|count+32 bit uint|count+16 bit int|count+16 bit uint|8 bit int null terminated|8 bit uint null terminated),edit
      mask CallbackString:
      | mquafifomask( 2, 2 );
      | |mquafifomask( 2, 2 );||||||||||||||||||||||
      mask Display:
      | disp('DSCP-200/300\nRS422/485\nSend Receive\nFIFO OUT');
      | port_label( 'input', 1, 'XMT1' );
      | port_label( 'input', 2, 'XMT2' );
      | port_label( 'output', 1, 'FIFO1' );
      | port_label( 'output', 2, 'FIFO2' );
  Modem Control : S-Function  InitFcn=mmodemcontrol(3)  FunctionName=modemcontrolqua  Parameters=slot, port, boardtype, rts, dtr, count  SFunctionModules='quatechinit'  EnableBusSupport=off  mask(DSCP-200/300 Modem Control){port=1, rts=on, dtr=on, slot=-1}
      mask prompts: slot "PCI slot: (-1 for autosearch)"
      mask help:
      | DSCP-200/300
      | Quatech
      | Modem Control
      mask init:
      | count = 0;
      | boardtype = 8;
      | [maskdisplay, count] = mmodemcontrol( 2, rts, dtr, boardtype, 0, 0 );
      | set_param( gcb, 'MaskDisplay', maskdisplay );
      mask Help: helpview(fullfile(docroot, 'mapfiles', 'xpc.map'), 'Quatech_MODEM_Control')
      mask StyleString: popup(1|2|3|4),checkbox,checkbox,edit
      mask Display: disp('DSCP-200/300\nQuatech\nModem Control');port_label('input',1,'RTS');port_label('input',2,'DTR');
  Modem Status : S-Function  FunctionName=modemstatusqua  Parameters=slot, port, boardtype, cts, dsr, ring, dcd, count, sampletime  SFunctionModules='quatechinit'  EnableBusSupport=off  mask(Modem Status){port=1, cts=on, dsr=on, ring=on, dcd=on, sampletime=-1, slot=-1}
      mask prompts: ring "RI:"; slot "PCI slot: (-1 for autosearch)"
      mask help:
      | DSCP-200/300
      | Quatech
      | Modem Status
      mask init:
      | count = 0;
      | boardtype = 8;
      | [maskdisplay, count] = mmodemstatus( 2, cts, dsr, ring, dcd, boardtype );
      | set_param( gcb, 'MaskDisplay', maskdisplay );
      mask Help: helpview(fullfile(docroot, 'mapfiles', 'xpc.map'), 'Quatech_MODEM_Status')
      mask StyleString: popup(1|2|3|4),checkbox,checkbox,checkbox,checkbox,edit,edit
      mask Display: disp('DSCP-200/300\nQuatech\nModem Status');port_label('output',1,'CTS');port_label('output',2,'DSR');port_label('output',3,'RI');port_label('output',4,'DCD');
